simulink model "fuzzy_TCLAB_toolbox_2015"  (R2015a)
settings: Solver=ode45  StartTime=0.0  StopTime=600  RelTol=1e-3
libraries: fuzblock x1
settings Model: CovHtmlReporting=off  Creator=Sergio  LastModifiedBy=Sergio
settings DataIOCC: SignalLoggingSaveFormat=ModelDataLogs
settings OptimizationCC: ExpressionDepthLimit=2147483647
settings DebuggingCC: UnderspecifiedInitializationDetection=Classic  MergeDetectMultiDrivingBlocksExec=none  SolverPrmCheckMsg=warning  FcnCallInpInsideContextMsg=EnableAllAsWarning  StateNameClashWarn=warning
settings GRTTargetCC: CombineOutputUpdateFcns=off  GRTInterface=on

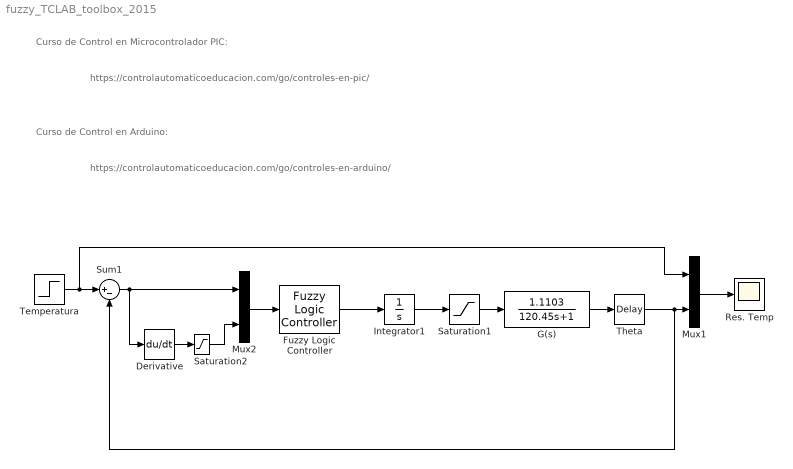
== system fuzzy_TCLAB_toolbox_2015 ==
  note: https://controlautomaticoeducacion.com/go/controles-en-pic/
  note: Curso de Control en Microcontrolador PIC:
  note: https://controlautomaticoeducacion.com/go/controles-en-arduino/
  note: Curso de Control en Arduino:
  Derivative : Derivative
  Fuzzy Logic Controller : fuzblock/Fuzzy Logic  Controller  FIS=PI_FUZZY
  G(s) : TransferFcn  Numerator=[1.1103]  Denominator=[120.45 1]
  Integrator1 : Integrator
  Mux1 : Mux  Inputs=2
  Mux2 : Mux  Inputs=2
  Res. Temp : Scope
      settings: TimeRange=auto  LimitDataPoints=on  MaxDataPoints=5000000  SaveToWorkspace=off  SaveName=ScopeData  YMin=-8.78666  YMax=79.07993  SampleTime=-1
  Saturation1 : Saturate  UpperLimit=100  LowerLimit=0
  Saturation2 : Saturate  UpperLimit=4  LowerLimit=-4
  Sum1 : Sum  Inputs=|+-
  Temperatura : Step  Time=0  After=50  SampleTime=0
  Theta : TransportDelay  DelayTime=12.78
  wires:
  Temperatura/1 -> Sum1/1, Mux1/1
  G(s)/1 -> Theta/1
  Theta/1 -> Mux1/2, Sum1/2
  Mux1/1 -> Res. Temp/1
  Mux2/1 -> Fuzzy Logic Controller/1
  Sum1/1 -> Mux2/1, Derivative/1
  Fuzzy Logic Controller/1 -> Integrator1/1
  Integrator1/1 -> Saturation1/1
  Saturation1/1 -> G(s)/1
  Saturation2/1 -> Mux2/2
  Derivative/1 -> Saturation2/1
